simulink model "two_discretization_formationcontrol"  (R2019a)
settings: Solver=VariableStepAuto  StartTime=0.0  StopTime=30  RelTol=1e-3
undefined symbols (not defined in the file): I, L
settings Model: Creator=DELL  LastModifiedBy=DELL

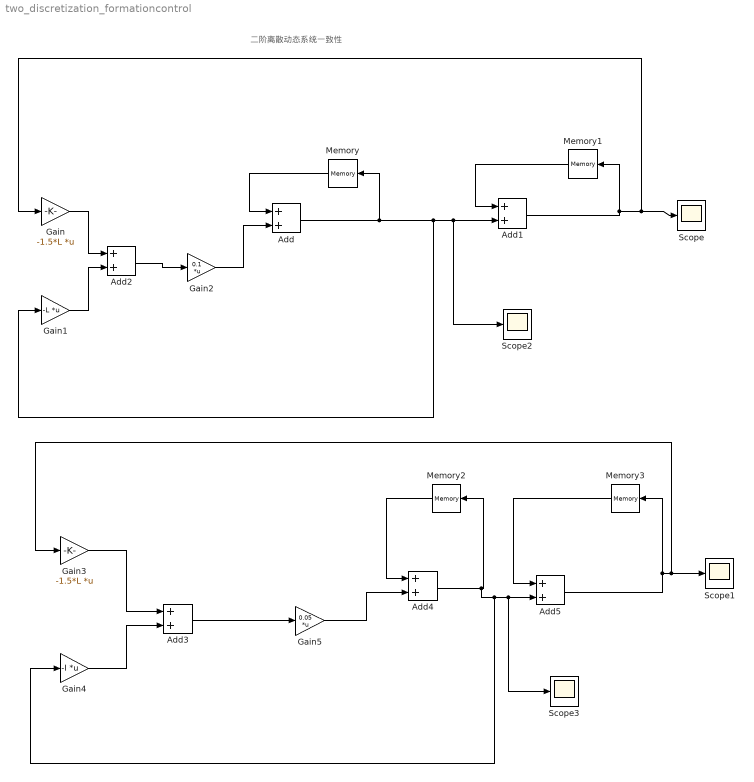
== system two_discretization_formationcontrol ==
  note: 二阶离散动态系统一致性
  Add{,1..5} (6 alike) : Sum
  Gain : Gain  Gain=-1.5*L  Multiplication=Matrix(K*u)
  Gain1 : Gain  Gain=-L  Multiplication=Matrix(K*u)
  Gain2 : Gain  Gain=0.1  Multiplication=Matrix(K*u)
  Gain3 : Gain  Gain=-1.5*L  Multiplication=Matrix(K*u)
  Gain4 : Gain  Gain=-I  Multiplication=Matrix(K*u)
  Gain5 : Gain  Gain=0.05  Multiplication=Matrix(K*u)
  Memory : Memory  InitialCondition=[2 1 4 0]
  Memory1 : Memory  InitialCondition=[20 10 40 0]
  Memory2 : Memory  InitialCondition=[2 1 4 0]
  Memory3 : Memory  InitialCondition=[20 10 40 0]
  Scope{,1..3} (4 alike) : Scope
  wires:
  Add/1 -> Memory/1, Gain1/1, Scope2/1, Add1/2
  Memory/1 -> Add/1
  Add1/1 -> Gain/1, Scope/1, Memory1/1
  Memory1/1 -> Add1/1
  Gain/1 -> Add2/1
  Gain1/1 -> Add2/2
  Add2/1 -> Gain2/1
  Gain2/1 -> Add/2
  Add3/1 -> Gain5/1
  Gain3/1 -> Add3/1
  Gain4/1 -> Add3/2
  Gain5/1 -> Add4/2
  Add4/1 -> Gain4/1, Scope3/1, Add5/2, Memory2/1
  Memory2/1 -> Add4/1
  Memory3/1 -> Add5/1
  Add5/1 -> Memory3/1, Gain3/1, Scope1/1
